simulink model "Testing_Interface"  (R2019b)
settings: Solver=ode1  StartTime=0.0  StopTime=60  FixedStep=0.005  RelTol=1e-3
InitFcn:
  | Testing_Interface_init()
values from neighbouring files (symbols this model uses):
  ALPHA_LIM_ENABLE = 1    [Testing_Interface_init.m]
  ALPHAMAX = pi/4    (= 0.785398163397)    [Testing_Interface_init.m]
  K_AMP = 1    [Testing_Interface_init.m]
  K_EC = Pr * N_pp / ( 4 * 1024 )    (= 2.27485440932e-05)    [Testing_Interface_init.m]
  K_EP = 2 * pi / ( 4 * 1024 )    (= 0.00153398078789)    [Testing_Interface_init.m]
  KF_Ts = 0.01    [Testing_Interface_init.m]
  X0 = [0; 0; pi; 0]    [Testing_Interface_init.m]
  X_LIM_ENABLE = 1    [Testing_Interface_init.m]
  XMAX = 0.35    [Testing_Interface_init.m]
undefined symbols (not defined in the file or in its folder): Humusoft, MF634, wcf, zetaf
libraries: sldrtlib x4, simulink_extras x2, sharedTrackingLibrary x1
settings Model: ExtModeTrigDuration=5000  Creator=Mfotoohi  LastModifiedBy=000
settings SolverCC: PositivePriorityOrder=on
settings DataIOCC: LimitDataPoints=on  SaveFormat=Array  ReturnWorkspaceOutputs=off
settings OptimizationCC: BooleanDataType=off  ExpressionDepthLimit=2147483647  InitFltsAndDblsToZero=on
settings DebuggingCC: SaveWithParameterizedLinksMsg=none  UnderspecifiedInitializationDetection=Classic  MergeDetectMultiDrivingBlocksExec=none  SolverPrmCheckMsg=warning  FcnCallInpInsideContextMsg=warning  StateNameClashWarn=warning  SFUnexpectedBacktrackingDiag=warning  SFNoUnconditionalDefaultTransitionDiag=warning  SFExecutionAtInitializationDiag=none  ArithmeticOperatorsInVariantConditions=warning
settings HardwareCC: ProdBitPerPointer=32  ProdBitPerSizeT=32  ProdBitPerPtrDiffT=32  ProdLargestAtomicFloat=None  ProdIntDivRoundTo=Undefined  ProdEndianess=Unspecified  ProdWordSize=32  ProdHWDeviceType=32-bit Generic
settings ModelReferenceCC: PropagateSignalLabelsOutOfModel=off
settings SFSimCC: SimUseLocalCustomCode=off  CustomCodeUndefinedFunction=UseInterfaceOnly
settings RTWCC: Description=Generic Real-Time Target  RTWUseLocalCustomCode=off
settings CodeAppCC: StateflowObjectComments=on
settings GRTTargetCC: TargetLangStandard=C89/C90 (ANSI)
settings ConfigComp: CovMetricSettings=dw  CovHtmlReporting=on  CovSaveCumulativeToWorkspaceVar=on  CovSaveSingleToWorkspaceVar=on  CovExternalEMLEnable=off

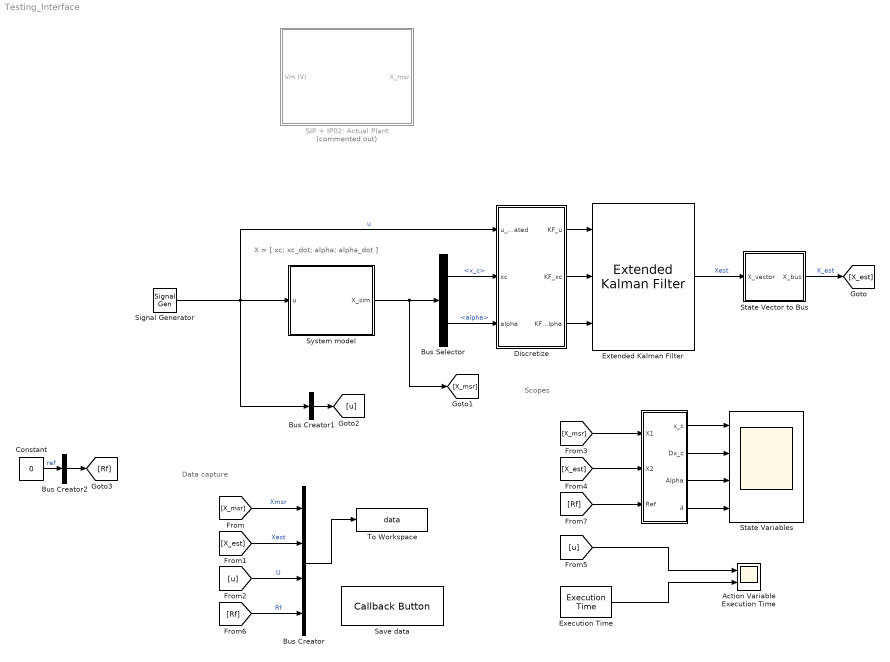
== system Testing_Interface ==
  note: Scopes
  note: X = [ xc; xc_dot; alpha; alpha_dot ]
  note: Data capture
  " " : Subsystem
  "Action Variable Execution Time " : Scope  NumInputPorts=2
  Bus Creator : BusCreator  Inputs=4
  Bus Creator1 : BusCreator  Inputs=1
  Bus Creator2 : BusCreator  Inputs=1
  Bus Selector : BusSelector  OutputSignals=x_c,alpha
  Constant : Constant  Value=0
  Discretize : Subsystem
  Execution Time : sldrtlib/Target Profiling/Execution Time  ShowTaskTimes=off
      settings: SourceProductName=Simulink Desktop Real-Time  SourceProductBaseCode=WT
  "Extended Kalman Filter " : sharedTrackingLibrary/Extended Kalman Filter  StateTransitionFcn=pendCartD  HasStateTransitionJacobianFcn=off  StateTransitionJacobianFcn=Jacobian  HasAdditiveProcessNoise=Additive  ProcessNoise=diag([1 5 1 5])  HasTimeVaryingProcessNoise=off  HasStateTransitionFcnExtraArgument=1  InitialState=X0  InitialStateCovariance=eye(4)  MeasurementFcn1=measure_x  HasMeasurementJacobianFcn1=off  HasMeasurementEnablePort1=off  HasAdditiveMeasurementNoise1=Additive  MeasurementNoise1=1  HasTimeVaryingMeasurementNoise1=off  HasMeasurementFcnExtraArgument1=0  MeasurementFcn2=measure_alpha  HasMeasurementJacobianFcn2=off  HasMeasurementEnablePort2=off  HasAdditiveMeasurementNoise2=Additive  MeasurementNoise2=1  HasTimeVaryingMeasurementNoise2=off  HasMeasurementFcnExtraArgument2=0  MeasurementFcn3=myMeasurementFcn  HasMeasurementJacobianFcn3=off  HasMeasurementEnablePort3=off  HasAdditiveMeasurementNoise3=Additive  MeasurementNoise3=1  HasTimeVaryingMeasurementNoise3=off  HasMeasurementFcnExtraArgument3=0  MeasurementFcn4=myMeasurementFcn  HasMeasurementJacobianFcn4=off  HasMeasurementEnablePort4=off  HasAdditiveMeasurementNoise4=Additive  MeasurementNoise4=1  HasTimeVaryingMeasurementNoise4=off  HasMeasurementFcnExtraArgument4=0  MeasurementFcn5=myMeasurementFcn  HasMeasurementJacobianFcn5=off  HasMeasurementEnablePort5=off  HasAdditiveMeasurementNoise5=Additive  MeasurementNoise5=1  HasTimeVaryingMeasurementNoise5=off  HasMeasurementFcnExtraArgument5=0  EnableMultirate=off  StateTransitionFcnSampleTime=1  MeasurementFcn1SampleTime=1  MeasurementFcn2SampleTime=1  MeasurementFcn3SampleTime=1  MeasurementFcn4SampleTime=1  MeasurementFcn5SampleTime=1  UseCurrentEstimator=on  OutputStateCovariance=off  DataType=double  SampleTime=KF_Ts  NumberOfMeasurements=2
      settings: SourceProductName=Automated Driving Toolbox  SourceProductBaseCode=DR
  SIP + IP02: Actual Plant : Subsystem  Commented=on
  Save data : CallbackButton  Tag=Save file  Description=save(saveFilePath, 'data');  ButtonText=Save
      settings: ClickFcn=save(saveFilePath, 'data');
  Signal Generator : SignalGenerator  WaveForm=sawtooth  Amplitude=4  Frequency=2  Units=rad/sec
  State Variables : Scope  NumInputPorts=4
  State Vector to Bus : Subsystem
  System model : Subsystem
  To Workspace : ToWorkspace  VariableName=data  SaveFormat=Timeseries  SampleTime=-1
  wires:
  Bus Selector/1 -> Discretize/2(xc)  "<x_c>"
  Bus Selector/2 -> Discretize/3(alpha)  "<alpha>"
  Discretize/1(KF_u) -> "Extended Kalman Filter "/1
  Discretize/2(KF_xc) -> "Extended Kalman Filter "/2
  Discretize/3(KF_alpha) -> "Extended Kalman Filter "/3
  "Extended Kalman Filter "/1 -> State Vector to Bus/1(X_vector)  "Xest"
  State Vector to Bus/1("X_bus ") -> [X_est]  "X_est"
  System model/1(X_sim) -> [X_msr], Bus Selector/1
  Bus Creator1/1 -> [u]
  [X_msr] -> " "/1(X1)
  [X_est] -> " "/2(X2)
  " "/1(x_c) -> State Variables/1
  [u] -> "Action Variable Execution Time "/1
  " "/2(Dx_c) -> State Variables/2
  " "/3(Alpha) -> State Variables/3
  " "/4(DAlpha) -> State Variables/4
  Execution Time/1 -> "Action Variable Execution Time "/2
  Signal Generator/1 -> Discretize/1(u_saturated), System model/1(u), Bus Creator1/1  "u"
  Constant/1 -> Bus Creator2/1  "ref"
  Bus Creator2/1 -> [Rf]
  [Rf] -> " "/3(Ref)
  [u] -> Bus Creator/3  "U"
  [X_est] -> Bus Creator/2  "Xest"
  Bus Creator/1 -> To Workspace/1
  [X_msr] -> Bus Creator/1  "Xmsr"
  [Rf] -> Bus Creator/4  "Rf"

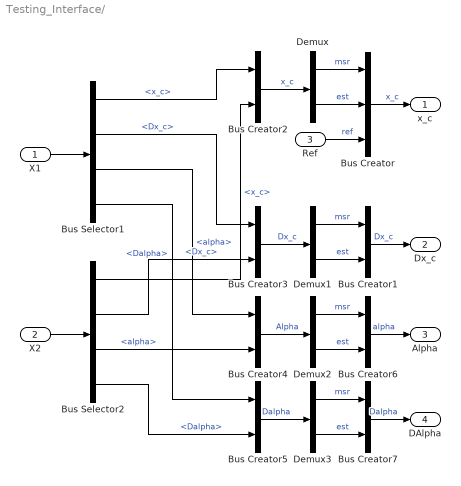
== system Testing_Interface/  ==
  X1 : Inport
  X2 : Inport  Port=2
  Ref : Inport  Port=3
  Bus Creator : BusCreator  Inputs=3
  Bus Creator{1..7} (7 alike) : BusCreator  Inputs=2
  Bus Selector1 : BusSelector  OutputSignals=x_c,Dx_c,alpha,Dalpha
  Bus Selector2 : BusSelector  OutputSignals=x_c,Dx_c,alpha,Dalpha
  Demux{,1..3} (4 alike) : Demux  Outputs=2
  x_c : Outport
  Dx_c : Outport  Port=2
  Alpha : Outport  Port=3
  DAlpha : Outport  Port=4
  wires:
  Ref/1 -> Bus Creator/3  "ref"
  Bus Creator1/1 -> Dx_c/1  "Dx_c"
  Demux2/1 -> Bus Creator6/1  "msr"
  Bus Creator5/1 -> Demux3/1  "Dalpha"
  Bus Creator7/1 -> DAlpha/1  "Dalpha"
  Demux3/2 -> Bus Creator7/2  "est"
  Bus Creator6/1 -> Alpha/1  "alpha"
  Demux3/1 -> Bus Creator7/1  "msr"
  Demux2/2 -> Bus Creator6/2  "est"
  Demux1/2 -> Bus Creator1/2  "est"
  Demux1/1 -> Bus Creator1/1  "msr"
  Bus Creator/1 -> x_c/1  "x_c"
  Demux/2 -> Bus Creator/2  "est"
  Demux/1 -> Bus Creator/1  "msr"
  X1/1 -> Bus Selector1/1
  X2/1 -> Bus Selector2/1
  Bus Selector2/1 -> Bus Creator2/2  "<x_c>"
  Bus Creator4/1 -> Demux2/1  "Alpha"
  Bus Selector2/4 -> Bus Creator5/2  "<Dalpha>"
  Bus Creator3/1 -> Demux1/1  "Dx_c"
  Bus Selector1/3 -> Bus Creator4/1  "<alpha>"
  Bus Selector1/2 -> Bus Creator3/1  "<Dx_c>"
  Bus Selector2/2 -> Bus Creator3/2  "<Dx_c>"
  Bus Creator2/1 -> Demux/1  "x_c"
  Bus Selector2/3 -> Bus Creator4/2  "<alpha>"
  Bus Selector1/4 -> Bus Creator5/1  "<Dalpha>"
  Bus Selector1/1 -> Bus Creator2/1  "<x_c>"

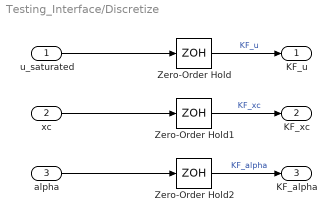
== system Testing_Interface/Discretize ==
  u_saturated : Inport
  xc : Inport  Port=2
  alpha : Inport  Port=3
  Zero-Order Hold : ZeroOrderHold  SampleTime=KF_Ts
  Zero-Order Hold1 : ZeroOrderHold  SampleTime=KF_Ts
  Zero-Order Hold2 : ZeroOrderHold  SampleTime=KF_Ts
  KF_u : Outport
  KF_xc : Outport  Port=2
  KF_alpha : Outport  Port=3
  wires:
  Zero-Order Hold2/1 -> KF_alpha/1  "KF_alpha"
  u_saturated/1 -> Zero-Order Hold/1
  alpha/1 -> Zero-Order Hold2/1
  Zero-Order Hold/1 -> KF_u/1  "KF_u"
  Zero-Order Hold1/1 -> KF_xc/1  "KF_xc"
  xc/1 -> Zero-Order Hold1/1

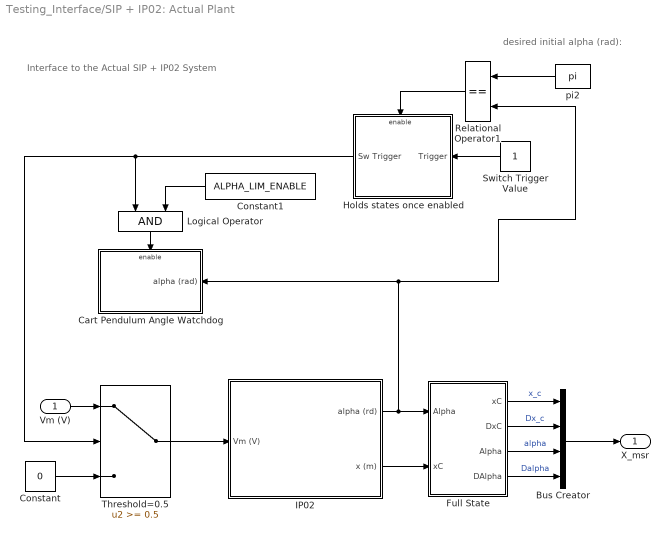
== system Testing_Interface/SIP + IP02: Actual Plant ==
  note: Interface to the Actual
      | SIP + IP02 System
  note: desired initial alpha (rad):
  Vm (V) : Inport
  Bus Creator : BusCreator  Inputs=4
  Cart Pendulum Angle Watchdog : Subsystem  TreatAsAtomicUnit=on
  Constant : Constant  Value=0
  Constant1 : Constant  Value=ALPHA_LIM_ENABLE  OutDataTypeStr=double
  "Full State " : Subsystem
  Holds states once enabled : Subsystem  TreatAsAtomicUnit=on
  "IP02 " : Subsystem
  Logical Operator : Logic
  Relational Operator1 : RelationalOperator  Operator===  RndMeth=Nearest  InputSameDT=on
  Switch Trigger Value : Constant
  Threshold=0.5 : Switch  Threshold=0.5  SaturateOnIntegerOverflow=on  InputSameDT=on
  pi2 : Constant  Value=pi
  "X_msr " : Outport  InitialOutput=0  VectorParamsAs1DForOutWhenUnconnected=off
  wires:
  "IP02 "/2(x (m)) -> "Full State "/2("xC ")
  Bus Creator/1 -> "X_msr "/1
  "Full State "/1(xC) -> Bus Creator/1  "x_c"
  "Full State "/2(DxC) -> Bus Creator/2  "Dx_c"
  "Full State "/3("Alpha ") -> Bus Creator/3  "alpha"
  "Full State "/4(DAlpha) -> Bus Creator/4  "Dalpha"
  Switch Trigger Value/1 -> Holds states once enabled/1(Trigger)
  Logical Operator/1 -> Cart Pendulum Angle Watchdog/Enable
  Constant1/1 -> Logical Operator/2
  Relational Operator1/1 -> Holds states once enabled/Enable
  Holds states once enabled/1(Sw Trigger) -> Logical Operator/1, Threshold=0.5/2
  pi2/1 -> Relational Operator1/1
  Constant/1 -> Threshold=0.5/3
  Vm (V)/1 -> Threshold=0.5/1
  Threshold=0.5/1 -> "IP02 "/1(Vm (V))
  "IP02 "/1(alpha (rd)) -> Relational Operator1/2, Cart Pendulum Angle Watchdog/1(alpha (rad)), "Full State "/1(Alpha)

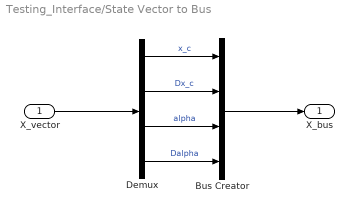
== system Testing_Interface/State Vector to Bus ==
  X_vector : Inport
  Bus Creator : BusCreator  Inputs=4
  Demux : Demux
  "X_bus " : Outport
  wires:
  Demux/3 -> Bus Creator/3  "alpha"
  Demux/1 -> Bus Creator/1  "x_c"
  Demux/2 -> Bus Creator/2  "Dx_c"
  Demux/4 -> Bus Creator/4  "Dalpha"
  Bus Creator/1 -> "X_bus "/1
  X_vector/1 -> Demux/1

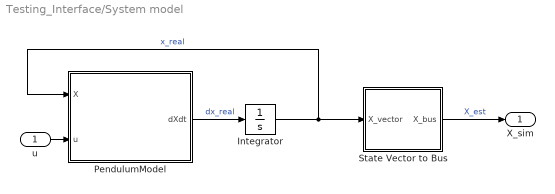
== system Testing_Interface/System model ==
  u : Inport
  Integrator : Integrator  InitialCondition=X0
  "PendulumModel " : MATLAB Function  TreatAsAtomicUnit=on
  State Vector to Bus : Subsystem
  X_sim : Outport
  wires:
  Integrator/1 -> State Vector to Bus/1(X_vector), "PendulumModel "/1(X)  "x_real"
  u/1 -> "PendulumModel "/2(u)
  "PendulumModel "/1(dXdt) -> Integrator/1  "dx_real"
  State Vector to Bus/1("X_bus ") -> X_sim/1  "X_est"

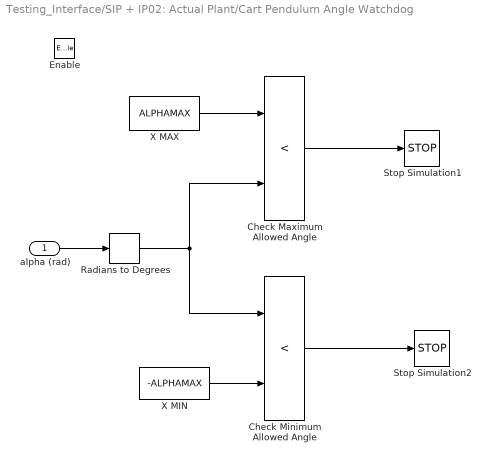
== system Testing_Interface/SIP + IP02: Actual Plant/Cart Pendulum Angle Watchdog ==
  alpha (rad) : Inport
  Enable : EnablePort
  Check Maximum Allowed Angle : RelationalOperator  Operator=<  RndMeth=Nearest  InputSameDT=on
  Check Minimum Allowed Angle : RelationalOperator  Operator=<  RndMeth=Nearest  InputSameDT=on
  Radians to Degrees : simulink_extras/Transformations/Radians to Degrees
  Stop Simulation1 : Stop
  Stop Simulation2 : Stop
  X MAX : Constant  Value=ALPHAMAX
  X MIN : Constant  Value=-ALPHAMAX
  wires:
  X MAX/1 -> Check Maximum Allowed Angle/1
  Check Minimum Allowed Angle/1 -> Stop Simulation2/1
  X MIN/1 -> Check Minimum Allowed Angle/2
  alpha (rad)/1 -> Radians to Degrees/1
  Check Maximum Allowed Angle/1 -> Stop Simulation1/1
  Radians to Degrees/1 -> Check Maximum Allowed Angle/2, Check Minimum Allowed Angle/1

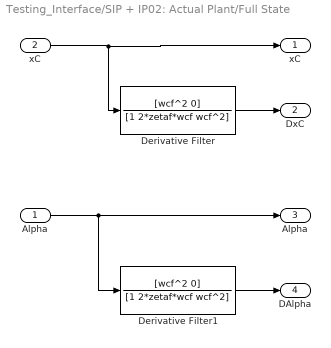
== system Testing_Interface/SIP + IP02: Actual Plant/Full State  ==
  Alpha : Inport
  "xC " : Inport  Port=2
  Derivative Filter : TransferFcn  Numerator=[wcf^2 0]  Denominator=[1 2*zetaf*wcf wcf^2]
  Derivative Filter1 : TransferFcn  Numerator=[wcf^2 0]  Denominator=[1 2*zetaf*wcf wcf^2]
  xC : Outport
  DxC : Outport  Port=2
  "Alpha " : Outport  Port=3
  DAlpha : Outport  Port=4
  wires:
  Alpha/1 -> Derivative Filter1/1, "Alpha "/1
  "xC "/1 -> xC/1, Derivative Filter/1
  Derivative Filter/1 -> DxC/1
  Derivative Filter1/1 -> DAlpha/1

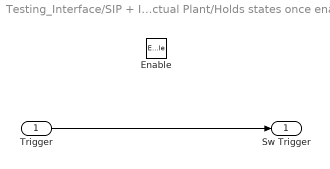
== system Testing_Interface/SIP + IP02: Actual Plant/Holds states once enabled ==
  Trigger : Inport  OutDataTypeStr=double
  Enable : EnablePort
  Sw Trigger : Outport  OutDataTypeStr=double  InitialOutput=[0]
  wires:
  Trigger/1 -> Sw Trigger/1

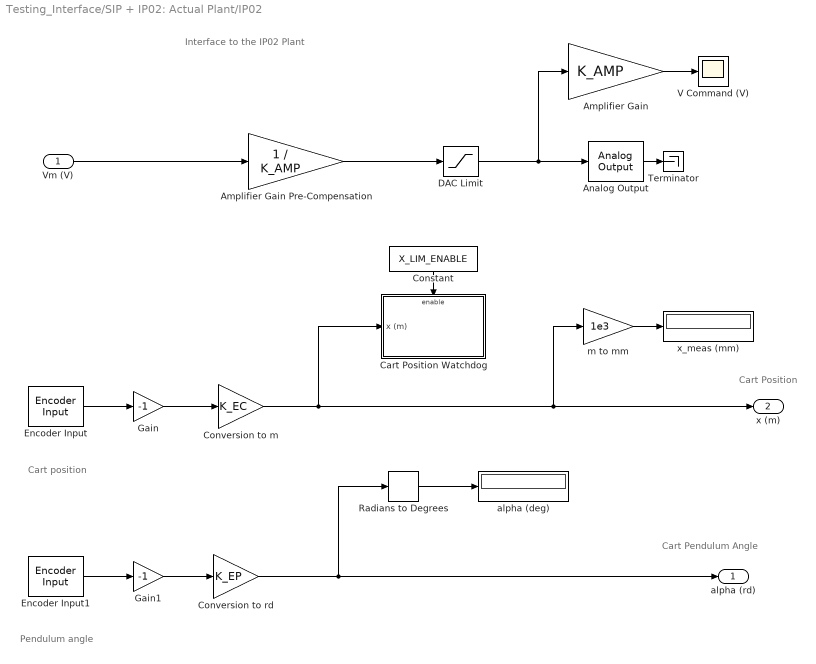
== system Testing_Interface/SIP + IP02: Actual Plant/IP02  ==
  note: Cart Pendulum Angle
  note: Cart Position
  note: Interface to the IP02 Plant
  note: Cart position
  note: Pendulum angle
  Vm (V) : Inport
  Amplifier Gain : Gain  Gain=K_AMP  SaturateOnIntegerOverflow=on  OutDataTypeStr=Inherit: Same as input  ParamDataTypeStr=Inherit: Same as input
  Amplifier Gain Pre-Compensation : Gain  Gain=1 / K_AMP  SaturateOnIntegerOverflow=on  OutDataTypeStr=Inherit: Same as input  ParamDataTypeStr=Inherit: Same as input
  Analog Output : sldrtlib/Analog Output  SampleTime=0.005  MaxMissedTicks=inf  ShowMissedTicks=on  YieldWhenWaiting=on  DrvName=Humusoft/MF634  DrvAddress=4294967295  DrvOptions=0  Channels=1  RangeMode=1  VoltRange=1  InitialValue=[]  FinalValue=0
      settings: AttributesFormatString=Humusoft\nMF634 [auto]  SourceProductName=Simulink Desktop Real-Time
  Cart Position Watchdog : Subsystem  TreatAsAtomicUnit=on
  Constant : Constant  Value=X_LIM_ENABLE
  Conversion to m : Gain  Gain=K_EC  SaturateOnIntegerOverflow=on  OutDataTypeStr=Inherit: Same as input  ParamDataTypeStr=Inherit: Same as input
  Conversion to rd : Gain  Gain=K_EP  SaturateOnIntegerOverflow=on  OutDataTypeStr=Inherit: Same as input  ParamDataTypeStr=Inherit: Same as input
  DAC Limit : Saturate  UpperLimit=10  LowerLimit=-10
  Encoder Input : sldrtlib/Encoder Input  SampleTime=0.005  MaxMissedTicks=inf  ShowMissedTicks=off  YieldWhenWaiting=on  DrvName=Humusoft/MF634  DrvAddress=4294967295  DrvOptions=0  Channels=1  QuadMode=3  IndexPulse=2  InputFilter=Inf  DataType=1
      settings: AttributesFormatString=Humusoft\nMF634 [auto]  SourceProductName=Simulink Desktop Real-Time
  Encoder Input1 : sldrtlib/Encoder Input  SampleTime=0.005  MaxMissedTicks=inf  ShowMissedTicks=off  YieldWhenWaiting=on  DrvName=Humusoft/MF634  DrvAddress=4294967295  DrvOptions=0  Channels=2  QuadMode=3  IndexPulse=2  InputFilter=Inf  DataType=1
      settings: AttributesFormatString=Humusoft\nMF634 [auto]  SourceProductName=Simulink Desktop Real-Time
  Gain : Gain  Gain=-1
  Gain1 : Gain  Gain=-1
  Radians to Degrees : simulink_extras/Transformations/Radians to Degrees
  Terminator : Terminator
  V Command (V) : Scope
  alpha (deg) : Display
      settings: Decimation=100
  m to mm : Gain  Gain=1e3  SaturateOnIntegerOverflow=on  OutDataTypeStr=Inherit: Same as input  ParamDataTypeStr=Inherit: Same as input
  x_meas (mm) : Display
      settings: Decimation=100
  alpha (rd) : Outport  InitialOutput=0
  x (m) : Outport  Port=2  InitialOutput=0
  wires:
  Gain/1 -> Conversion to m/1
  Conversion to m/1 -> Cart Position Watchdog/1(x (m)), x (m)/1, m to mm/1
  Amplifier Gain Pre-Compensation/1 -> DAC Limit/1
  m to mm/1 -> x_meas (mm)/1
  Gain1/1 -> Conversion to rd/1
  Radians to Degrees/1 -> alpha (deg)/1
  Conversion to rd/1 -> Radians to Degrees/1, alpha (rd)/1
  Constant/1 -> Cart Position Watchdog/Enable
  DAC Limit/1 -> Analog Output/1, Amplifier Gain/1
  Vm (V)/1 -> Amplifier Gain Pre-Compensation/1
  Amplifier Gain/1 -> V Command (V)/1
  Encoder Input1/1 -> Gain1/1
  Encoder Input/1 -> Gain/1
  Analog Output/1 -> Terminator/1

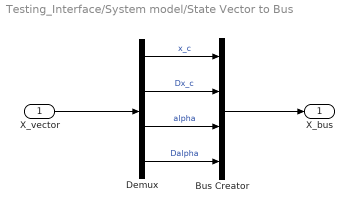
== system Testing_Interface/System model/State Vector to Bus ==
  X_vector : Inport
  Bus Creator : BusCreator  Inputs=4
  Demux : Demux
  "X_bus " : Outport
  wires:
  Demux/3 -> Bus Creator/3  "alpha"
  Demux/1 -> Bus Creator/1  "x_c"
  Demux/2 -> Bus Creator/2  "Dx_c"
  Demux/4 -> Bus Creator/4  "Dalpha"
  Bus Creator/1 -> "X_bus "/1
  X_vector/1 -> Demux/1

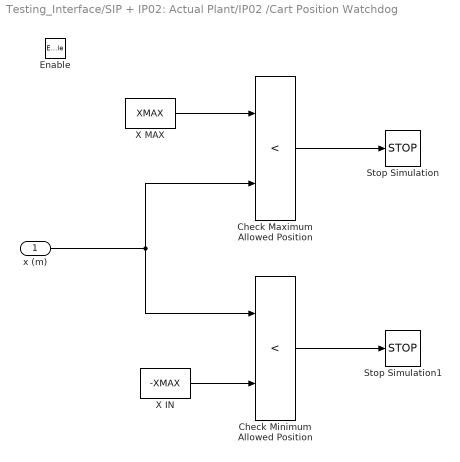
== system Testing_Interface/SIP + IP02: Actual Plant/IP02 /Cart Position Watchdog ==
  x (m) : Inport
  Enable : EnablePort
  Check Maximum Allowed Position : RelationalOperator  Operator=<  RndMeth=Nearest  InputSameDT=on
  Check Minimum Allowed Position : RelationalOperator  Operator=<  RndMeth=Nearest  InputSameDT=on
  Stop Simulation : Stop
  Stop Simulation1 : Stop
  X IN : Constant  Value=-XMAX
  X MAX : Constant  Value=XMAX
  wires:
  Check Maximum Allowed Position/1 -> Stop Simulation/1
  x (m)/1 -> Check Minimum Allowed Position/1, Check Maximum Allowed Position/2
  X IN/1 -> Check Minimum Allowed Position/2
  Check Minimum Allowed Position/1 -> Stop Simulation1/1
  X MAX/1 -> Check Maximum Allowed Position/1

== matlab function Testing_Interface/System model/PendulumModel  ==
  data: X input; u input; dXdt output
function dXdt = pendCartC(X,u)
%PENDCARTC
%    DXDT = PENDCARTC(IN1,U)

%    This function was generated by the Symbolic Math Toolbox version 8.4.
%    19-May-2020 20:15:22

X2 = X(2,:);
X3 = X(3,:);
X4 = X(4,:);
t2 = cos(X3);
t3 = sin(X3);
t4 = X4.^2;
t5 = t2.^2;
t6 = t5.*4.565807400625001e-4;
t7 = t6-3.005650706948956e-3;
t8 = 1.0./t7;
dXdt = [X2;t8.*(X2.*(-5.665253057117538e-6)+u.*5.387661376655595e-7+X4.*t2.*5.3763908601e-9+t2.*t3.*4.695776235861861e-7+t3.*t4.*1.074185854609239e-8).*(-9.53848061542277e+3);X4;t8.*(X4.*1.57714169184e-7+t3.*1.377486248645154e-5-X2.*t2.*2.524516833955624e-5+t2.*u.*2.40081805770912e-6+t2.*t3.*t4.*4.786723991704242e-8).*9.53848061542277e+3];
